simulink model "uGrid_1PH_hd_ATD2"  (R2018a)
settings: Solver=VariableStepAuto  StartTime=0.0  StopTime=0.8  FixedStep=1e-6  MaxStep=1e-4  RelTol=1e-3
PreLoadFcn:
  | SimulinkInit
InitFcn:
  | SimulinkInit
StopFcn:
  | EndingScript
values from neighbouring files (symbols this model uses):
  Ad = sysd.A    [SimulinkInit.m]
  Bd = sysd.B    [SimulinkInit.m]
  C1 = Cd(2,:)    [SimulinkInit.m]
  C10 = Cd(1,:)    [SimulinkInit.m]
  C11 = Cd(2,:)    [SimulinkInit.m]
  C12 = Cd(3,:)    [SimulinkInit.m]
  C2 = Cd(3,:)    [SimulinkInit.m]
  C3 = Cd(4,:)    [SimulinkInit.m]
  C4 = Cd(1,:)    [SimulinkInit.m]
  C5 = Cd(3,:)    [SimulinkInit.m]
  C6 = Cd(4,:)    [SimulinkInit.m]
  C7 = Cd(1,:)    [SimulinkInit.m]
  C8 = Cd(2,:)    [SimulinkInit.m]
  C9 = Cd(4,:)    [SimulinkInit.m]
  Cd = sysd.C    [SimulinkInit.m]
  T1 = 0.4    [parametros_BIO.m]
  T2 = 1    [parametros_BIO.m]
  T3 = 15    [parametros_BIO.m]
  T4 = 2.5    [parametros_BIO.m]
  T5 = 3.3    [parametros_BIO.m]
  Tao1 = 0.5    [SimulinkInit.m]
  tm = 1e-4    (= 0.0001)    [SimulinkInit.m]
undefined symbols (not defined in the file or in its folder): F1, F10, F11, F12, F2, F3, F4, F5, F6, F7, F8, F9, G, GF, H1, H10, H11, H12, H2, H3, H4, H5, H6, H7, H8, H9, Ion, K10U, K11U, K12U, K1U, K2U, K3U, K4U, K5U, K6U, K7U, K8U, K9U, Lithium, ss1, ss2, T10, T11, T12, T6, T7, T8, T9
libraries: powerlib x59, dsparch4 x17, truetime x12, powerlib_meascontrol x6, simulink x2, dspstat3 x2, dspfdesign x1, electricdrivelib x1
(part 3 of 3)

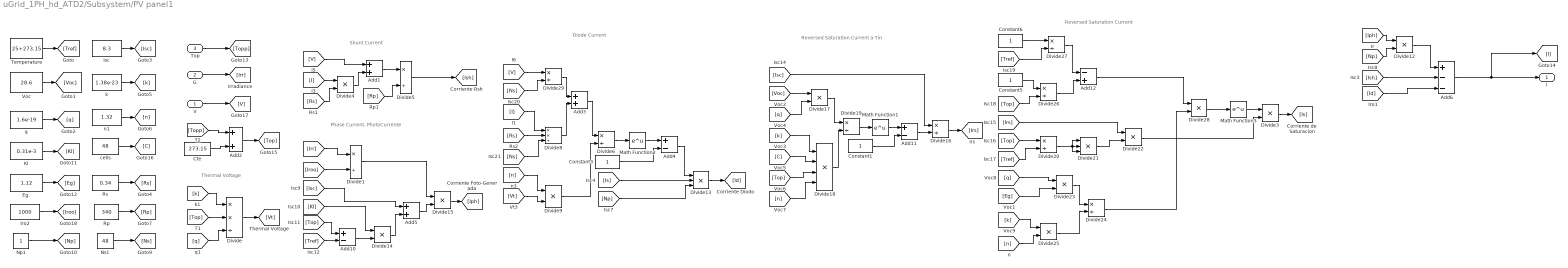
== system uGrid_1PH_hd_ATD2/Subsystem/PV panel1 ==
  note: Thermal Voltage
  note: Shunt Current
  note: Phase Current- PhotoCurrente
  note: Diode Current
  note: Reversed Saturation Current a Tin
  note: Reversed Saturation Current
  V : Inport
  G : Inport  Port=2
  Top : Inport  Port=3
  Add{1..3,5} (4 alike) : Sum
  Add10 : Sum  Inputs=+-
  Add11 : Sum  Inputs=+-
  Add12 : Sum  Inputs=-+
  Add4 : Sum  Inputs=+-
  Add6 : Sum  Inputs=+--
  Constant{1,3,5..6} (4 alike) : Constant
  Cte : Constant  Value=273.15
  Divide : Product  Inputs=**/
  Divide{1,5..6,16,19..20,24,26..27,29} (10 alike) : Product  Inputs=*/
  Divide{3..4,9,12,14..15,17,22..23,25,28} (11 alike) : Product  Inputs=**
  Divide13 : Product  Inputs=***
  Divide18 : Product  Inputs=****
  Divide21 : Product  Inputs=***
  Divide8 : Product  Inputs=**/
  Eg. : Constant  Value=1.12
  Iro2 : Constant  Value=1000
  Isc : Constant  Value=8.3
  KI : Constant  Value=0.31e-3
  Math Function1 : Math  SaturateOnIntegerOverflow=on
  Math Function2 : Math  SaturateOnIntegerOverflow=on
  Math Function3 : Math  SaturateOnIntegerOverflow=on
  Np1 : Constant
  Ns1 : Constant  Value=48
  Rp : Constant  Value=340
  Rs : Constant  Value=0.34
  Temperature : Constant  Value=25+273.15
  Voc : Constant  Value=28.6
  cells : Constant  Value=48
  k : Constant  Value=1.38e-23
  n1 : Constant  Value=1.32
  q : Constant  Value=1.6e-19
  I : Outport
  wires:
  Temperature/1 -> [Tref]
  Voc/1 -> [Voc]
  q/1 -> [q]
  Isc/1 -> [Isc]
  k/1 -> [k]
  n1/1 -> [n]
  [k] -> Divide/1
  [Top] -> Divide/2
  [q] -> Divide/3
  Divide/1 -> [Vt]
  Divide3/1 -> [Is]
  [Ish] -> Add6/2
  Add6/1 -> I/1, [I]
  [I] -> Divide8/1
  [Rs] -> Divide8/2
  Divide8/1 -> Add3/2
  [n] -> Divide9/1
  [Vt] -> Divide9/2
  Divide9/1 -> Divide6/2
  Add3/1 -> Divide6/1
  Divide6/1 -> Math Function2/1
  Math Function2/1 -> Add4/1
  Add4/1 -> Divide13/1
  [Is] -> Divide13/2
  Divide13/1 -> [Id]
  Divide4/1 -> Add1/2
  Add1/1 -> Divide5/1
  [Rp] -> Divide5/2
  Divide5/1 -> [Ish]
  [Rs] -> Divide4/2
  [I] -> Divide4/1
  KI/1 -> [KI]
  Eg./1 -> [Eg]
  [V] -> Add1/1
  [Np] -> Divide13/3
  [Iph] -> Divide12/1
  [Np] -> Divide12/2
  Divide12/1 -> Add6/1
  [Isc] -> Add5/1
  [Top] -> Add10/1
  [Tref] -> Add10/2
  Add10/1 -> Divide14/2
  [KI] -> Divide14/1
  [Voc] -> Divide17/1
  [q] -> Divide17/2
  [k] -> Divide18/1
  [C] -> Divide18/2
  [Top] -> Divide18/3
  [n] -> Divide18/4
  Divide17/1 -> Divide19/1
  Divide18/1 -> Divide19/2
  Divide19/1 -> Math Function1/1
  Constant1/1 -> Add11/2
  Math Function1/1 -> Add11/1
  Add11/1 -> Divide16/2
  Divide16/1 -> [Irs]
  [Tref] -> Divide20/2
  [Top] -> Divide20/1
  Divide20/1 -> Divide21/2, Divide21/1, Divide21/3
  Divide21/1 -> Divide22/2
  [Irs] -> Divide22/1
  [q] -> Divide23/1
  Divide23/1 -> Divide24/1
  [k] -> Divide25/1
  [n] -> Divide25/2
  Divide25/1 -> Divide24/2
  Constant5/1 -> Divide26/1
  [Top] -> Divide26/2
  Constant6/1 -> Divide27/1
  [Tref] -> Divide27/2
  Divide27/1 -> Add12/1
  Divide26/1 -> Add12/2
  Add12/1 -> Divide28/1
  Divide24/1 -> Divide28/2
  Divide28/1 -> Math Function3/1
  Divide29/1 -> Add3/1
  [Ns] -> Divide29/2
  [V] -> Divide29/1
  [Ns] -> Divide8/3
  Divide14/1 -> Add5/2
  Add5/1 -> Divide15/2
  Divide15/1 -> [Iph]
  V/1 -> [V]
  G/1 -> [Irr]
  Top/1 -> [Topp]
  cells/1 -> [C]
  [Id] -> Add6/3
  Cte/1 -> Add2/2
  Add2/1 -> [Top]
  [Topp] -> Add2/1
  [Irr] -> Divide1/1
  [Iroo] -> Divide1/2
  Divide1/1 -> Divide15/1
  Iro2/1 -> [Iroo]
  Rs/1 -> [Rs]
  Rp/1 -> [Rp]
  Ns1/1 -> [Ns]
  Np1/1 -> [Np]
  Constant3/1 -> Add4/2
  [Isc] -> Divide16/1
  Math Function3/1 -> Divide3/1
  Divide22/1 -> Divide3/2
  [Eg] -> Divide23/2

== system uGrid_1PH_hd_ATD2/1Ph_Inverter_bio/Subsystem/Steper1 ==
  In1 : Inport
  Product : Product
  Step : Step  Time=st_time  SampleTime=samp_f
  Out1 : Outport
  wires:
  Step/1 -> Product/2
  In1/1 -> Product/1
  Product/1 -> Out1/1

== system uGrid_1PH_hd_ATD2/1Ph_Inverter_bio/Subsystem/Steper3 ==
  In1 : Inport
  Product : Product
  Step : Step  Time=st_time  SampleTime=samp_f
  Out1 : Outport
  wires:
  Product/1 -> Out1/1
  In1/1 -> Product/1
  Step/1 -> Product/2

== system uGrid_1PH_hd_ATD2/1Ph_Inverter_diesel/Subsystem/Steper1 ==
  In1 : Inport
  Product : Product
  Step : Step  Time=st_time  SampleTime=samp_f
  Out1 : Outport
  wires:
  Product/1 -> Out1/1
  In1/1 -> Product/1
  Step/1 -> Product/2

== system uGrid_1PH_hd_ATD2/1Ph_Inverter_diesel/Subsystem/Steper3 ==
  In1 : Inport
  Product : Product
  Step : Step  Time=st_time  SampleTime=samp_f
  Out1 : Outport
  wires:
  Step/1 -> Product/2
  In1/1 -> Product/1
  Product/1 -> Out1/1

== matlab function uGrid_1PH_hd_ATD2/1Ph_Inverter_diesel/Subsystem/not_pwm ==
  data: u input; y output
function y = fcn(u)
%#codegen

if(u==0 || u<0)
    a=15;
else
    a=0;
end;

y = a;

== matlab function uGrid_1PH_hd_ATD2/1Ph_Inverter_bio/Subsystem/not_pwm ==
  data: u input; y output
function y = fcn(u)
%#codegen

if(u==0 || u<0)
    a=15;
else
    a=0;
end;

y = a;

== matlab function uGrid_1PH_hd_ATD2/LinearProg ==
  data: P_load input; Pbo output; P_e_alt input; kb input; kd input; PdMax input; PbMax input; Pdo output; P_e_alt_min input
function [Pbo, Pdo] = fcn(P_load, P_e_alt, kb, kd, PdMax, PbMax, P_e_alt_min)

% P_load es la potencia que se requiere en la carga.

% P_e_alt es la potencia estimada de generacion de las energias
% alternativas

% kb y kd son los pesos de las funcion de costo.

% las salidas son las potencias optimas para bio y diesel

Pb=0;
Pd=0;

D_P_e_alt = P_e_alt - P_e_alt_min % superaavit de energia alternativa.

flagDelt = 0;

if(D_P_e_alt >= P_load)
    flagDelt = 1;
end
   

if(flagDelt==0)
    P_trad = P_load - D_P_e_alt;
    % flag: variable que indica si tiene sentido evaluar los
    % if's que se encuentran mas adelante. es decir, si flag = 0 
    % despues del primer if entonces NO se le esta pidiendo al sistema
    % mas potencia de la que puede generar y portanto el problema de 
    % optimizacion lineal tiene sentido.
    % entonces 
    flag=0;

    if(P_trad>PdMax+PbMax)
        Pd=PdMax;
        Pb=PbMax;
        flag=1;
    end

    % si ambas energias tienen el mismo factor de costo.
    if(kd==kb && flag==0)
        Pb=P_trad/2;
        Pd=P_trad/2;
    end

    % si la energia diesel es mas cara que la biomasa.
    if(kd>kb && flag==0)
        if(P_trad<=PbMax)
            Pb=P_trad;
            Pd=0;
        else
            Pb=PbMax;
            Pd=P_trad-PbMax;
        end
    end

    % si la biomasa es mas cara que la diesel.
    if(kd<kb && flag==0)
        if(P_trad<=PdMax)
            Pd=P_trad;
            Pb=0;
        else
            Pd=PdMax;
            Pb=P_trad-PdMax;
        end
    end
end

Pbo=Pb;
Pdo=Pd;

== matlab function uGrid_1PH_hd_ATD2/MPC Controller/MPC_MatCalc1 ==
  data: ref input; PQ input; Hv output; F output; A output; lb output; ub output; lbA output; ubA output; Du input; MPCout input; G input; GF input
function [Hv, F, A, lb, ub, lbA, ubA] = MPC(ref, PQ, Du, MPCout, G, GF)

%%parametros del MPC


p = 100; % horizonte de prediccion
Nu = 100; % horizonte de control


%% Calculo de la salida de control.

H = G'*G+eye(2*Nu)*3000; % parte cuadratica del qp

ym = [ ones(p, 1)*PQ(1); ones(p, 1)*PQ(2) ]; % vector de la medida de tempearatura actual.

w = [ ones(p, 1)*ref(1); ones(p, 1)*ref(2) ]; % vector señal setpoint.

L = GF*Du+ym; % respuesta libre.

F = 2*(L-w)'*G; % parte lineal del problema qp.

A = zeros(1, 4*Nu*Nu);

lbA = zeros(1, 2*Nu);

ubA = zeros(1, 2*Nu);

Hv = M2V(H);

hip = HiBound(MPCout(1), 600, 10);
hiq = HiBound(MPCout(2), 5000, 1000);

lop = LowBound(MPCout(1), -100, -10);
loq = LowBound(MPCout(2), -100, -1000);

lb = [ones(1, Nu)*lop ones(1, Nu)*loq];
ub = [ones(1, Nu)*hip ones(1, Nu)*hiq];
end

% el control mpc implementado halla mediante programacion cuadratica
% los delta de u optimos deacuerdo a la funcion de coste. por este motivo
% es necesario implementar una logica adicional que permita limitar
% los valores de u (la salida) ya que estos no se manupilan directamente
% en el problema de programacion cuadratica.

% esta logica se implementan en las dos funciones locales que se encuentran
% a continuacion. una funcion define el limite superior y otra funcion para
% definir el limite inferior de los deltas de u deacuerdo al valor actual
% de u para asegurar que tanto los deltas de u como el valor de u esten
% limitados.
% esta funcion solo es correcta si max y Dmax son valores positivos.
function y = HiBound(X, max, Dmax)
    if(X>=0) % si la potencia X es positiva:
        if(max >= X)% si X no ha superado la potencia maxima:
            if(max-X >= Dmax) % si la distancia supera el cambio maximo deseado
                r = Dmax;
            else % si es menor al cambio maximo deseado
                r = max-X;
            end
        else % si X supera la potencia maxima deseada
            r = 0; % el delta maximo es 0 para que no se incremente mas.
        end
    else % si la potencia X es negativa, el incremento maximo es
        r = Dmax;
    end
    y = r;
end

% esta funcion para el lower bound se penso para trbajar con valores
% negativos. si min y Dmin no es negativo la funcion no funciona
% correctamente.
function y = LowBound(X, minv, Dmin)
    if(X<=0) % si la potencia X esta en el cuadrante inferior:
        if(minv <= X)% si X es mayor que la potencia minima:
            if(minv-X <= Dmin) % si la distancia supera el cambio maximo deseado
                r = Dmin;
            else % si es mayor al cambio maximo deseado
                r = minv-X;
            end
        else % si X es menor la potencia maxima deseada
            r = 0; % el delta maximo es 0 para que no se decremente mas.
        end
    else % si la potencia X es positiva, el decremento maximo es
        r = Dmin;
    end
    y = r;
end

== matlab function uGrid_1PH_hd_ATD2/MPC Controller/MPC_OutLogic1 ==
  data: MPCout output; duv input; Duv output
function [MPCout, Duv] = MPC_out_Logic(duv)

%%parametros del MPC
Nu = 100; % horizonte de control.


%% variables del MPC
persistent Du; % deltas de u 
persistent out; % salida actual del conrolador MPC.

if isempty(Du) % inicializacion de los deltas de uu
    Du = zeros(2*Nu, 1);
end

if isempty(out) % inicializaion de la salida del controlador MPC
    out = [0; 0];
end


du = [duv(1), duv(Nu+1)];


Du = [du(1); Du(1:Nu-1); du(2); Du(Nu+1:end-1)];% actualizar historial deltas de u.

out = [ out(1)+du(1); out(2)+du(2) ]; %calcular salida del controlador.

MPCout = out;
Duv = Du;

== matlab function uGrid_1PH_hd_ATD2/MPC Controller/MPC_MatCalc ==
  data: ref input; PQ input; Hv output; F output; A output; lb output; ub output; lbA output; ubA output; Du input; MPCout input; G input; GF input
function [Hv, F, A, lb, ub, lbA, ubA] = MPC(ref, PQ, Du, MPCout, G, GF)

%%parametros del MPC


p = 100; % horizonte de prediccion
Nu = 100; % horizonte de control


%% Calculo de la salida de control.

H = G'*G+eye(2*Nu)*3000; % parte cuadratica del qp

ym = [ ones(p, 1)*PQ(1); ones(p, 1)*PQ(2) ]; % vector de la medida de tempearatura actual.

w = [ ones(p, 1)*ref(1); ones(p, 1)*ref(2) ]; % vector señal setpoint.

L = GF*Du+ym; % respuesta libre.

F = 2*(L-w)'*G; % parte lineal del problema qp.

A = zeros(1, 4*Nu*Nu);

lbA = zeros(1, 2*Nu);

ubA = zeros(1, 2*Nu);

Hv = M2V(H);

hip = HiBound(MPCout(1), 600, 10);
hiq = HiBound(MPCout(2), 5000, 1000);

lop = LowBound(MPCout(1), -100, -10);
loq = LowBound(MPCout(2), -100, -1000);

lb = [ones(1, Nu)*lop ones(1, Nu)*loq];
ub = [ones(1, Nu)*hip ones(1, Nu)*hiq];
end

% el control mpc implementado halla mediante programacion cuadratica
% los delta de u optimos deacuerdo a la funcion de coste. por este motivo
% es necesario implementar una logica adicional que permita limitar
% los valores de u (la salida) ya que estos no se manupilan directamente
% en el problema de programacion cuadratica.

% esta logica se implementan en las dos funciones locales que se encuentran
% a continuacion. una funcion define el limite superior y otra funcion para
% definir el limite inferior de los deltas de u deacuerdo al valor actual
% de u para asegurar que tanto los deltas de u como el valor de u esten
% limitados.
% esta funcion solo es correcta si max y Dmax son valores positivos.
function y = HiBound(X, max, Dmax)
    if(X>=0) % si la potencia X es positiva:
        if(max >= X)% si X no ha superado la potencia maxima:
            if(max-X >= Dmax) % si la distancia supera el cambio maximo deseado
                r = Dmax;
            else % si es menor al cambio maximo deseado
                r = max-X;
            end
        else % si X supera la potencia maxima deseada
            r = 0; % el delta maximo es 0 para que no se incremente mas.
        end
    else % si la potencia X es negativa, el incremento maximo es
        r = Dmax;
    end
    y = r;
end

% esta funcion para el lower bound se penso para trbajar con valores
% negativos. si min y Dmin no es negativo la funcion no funciona
% correctamente.
function y = LowBound(X, minv, Dmin)
    if(X<=0) % si la potencia X esta en el cuadrante inferior:
        if(minv <= X)% si X es mayor que la potencia minima:
            if(minv-X <= Dmin) % si la distancia supera el cambio maximo deseado
                r = Dmin;
            else % si es mayor al cambio maximo deseado
                r = minv-X;
            end
        else % si X es menor la potencia maxima deseada
            r = 0; % el delta maximo es 0 para que no se decremente mas.
        end
    else % si la potencia X es positiva, el decremento maximo es
        r = Dmin;
    end
    y = r;
end

== matlab function uGrid_1PH_hd_ATD2/MPC Controller/MPC_OutLogic ==
  data: MPCout output; duv input; Duv output
function [MPCout, Duv] = MPC_out_Logic(duv)

%%parametros del MPC
Nu = 100; % horizonte de control.


%% variables del MPC
persistent Du; % deltas de u 
persistent out; % salida actual del conrolador MPC.

if isempty(Du) % inicializacion de los deltas de uu
    Du = zeros(2*Nu, 1);
end

if isempty(out) % inicializaion de la salida del controlador MPC
    out = [0; 0];
end


du = [duv(1), duv(Nu+1)];


Du = [du(1); Du(1:Nu-1); du(2); Du(Nu+1:end-1)];% actualizar historial deltas de u.

out = [ out(1)+du(1); out(2)+du(2) ]; %calcular salida del controlador.

MPCout = out;
Duv = Du;

== matlab function uGrid_1PH_hd_ATD2/1Ph_Inverter_bio1/not_pwm ==
  data: u input; y output
function y = fcn(u)
%#codegen

if(u==0 || u<0)
    a=15;
else
    a=0;
end;

y = a;

== matlab function uGrid_1PH_hd_ATD2/BioMassGenerator/Subsystem1/MATLAB Function ==
  data: w input; Pe input; Tm output
function Tm = fcn(w, Pe)

max_torq=30000;

if w>0
    Tm = Pe/w;
else
    Tm = max_torq;
end

== matlab function uGrid_1PH_hd_ATD2/LinearProg1 ==
  data: Q_load input; Qbo output; Q_e_alt input; kb input; kd input; QdMax input; QbMax input; Qdo output; Q_e_alt_min input
function [Qbo, Qdo] = fcn(Q_load, Q_e_alt, kb, kd, QdMax, QbMax, Q_e_alt_min)

% Q_load es la Qotencia que se requiere en la carga.

% Q_e_alt es la Qotencia estimada de generacion de las energias
% alternativas

% kb y kd son los Qesos de las funcion de costo.

% las salidas son las Qotencias oQtimas Qara bio y diesel

Qb=0;
Qd=0;

D_Q_e_alt = Q_e_alt - Q_e_alt_min % suQeraavit de energia alternativa.

flagDelt = 0;

if(D_Q_e_alt >= Q_load)
    flagDelt = 1;
end
   

if(flagDelt==0)
    Q_trad = Q_load - D_Q_e_alt;
    % flag: variable que indica si tiene sentido evaluar los
    % if's que se encuentran mas adelante. es decir, si flag = 0 
    % desQues del Qrimer if entonces NO se le esta Qidiendo al sistema
    % mas Qotencia de la que Quede generar y Qortanto el Qroblema de 
    % oQtimizacion lineal tiene sentido.
    % entonces 
    flag=0;

    if(Q_trad>QdMax+QbMax)
        Qd=QdMax;
        Qb=QbMax;
        flag=1;
    end

    % si ambas energias tienen el mismo factor de costo.
    if(kd==kb && flag==0)
        Qb=Q_trad/2;
        Qd=Q_trad/2;
    end

    % si la energia diesel es mas cara que la biomasa.
    if(kd>kb && flag==0)
        if(Q_trad<=QbMax)
            Qb=Q_trad;
            Qd=0;
        else
            Qb=QbMax;
            Qd=Q_trad-QbMax;
        end
    end

    % si la biomasa es mas cara que la diesel.
    if(kd<kb && flag==0)
        if(Q_trad<=QdMax)
            Qd=Q_trad;
            Qb=0;
        else
            Qd=QdMax;
            Qb=Q_trad-QdMax;
        end
    end
end

Qbo=Qb;
Qdo=Qd;

== matlab function uGrid_1PH_hd_ATD2/FRACASO/MATLAB Function4 ==
  data: r input; rol output; r1 input
function rol = fcn(r,r1)%u1,u2,ym1,ym2)
Th_det = 6.5e-8;
Th_det=0.1;  %2.5

m=r-r1;
if m>0
    Th_det=0.1;  %2.5
elseif m<0 && r<=0.1
    Th_det=0.9; 
end


% sys=tf(1,[0.001 1]);


if r >=Th_det
    rol=1;
else
    rol=0;
end

== matlab function uGrid_1PH_hd_ATD2/FRACASO/MATLAB Function3 ==
  data: y_hat input; rol output; y_m input; norm_rd output; tiempo input
function [rol,norm_rd] = fcn(y_hat,y_m,tiempo)%u1,u2,ym1,ym2)
Th_det = 6.5e-8;
Th_det=0.07;%2.3e-2; %Funciona bien si los pulsos no estan tan separados
Th_det_up=1;  %2.5 2.25
Th_det_down=-1;
if tiempo >=0.0015 && tiempo <=0.35
    Th_det_up=2.23e-2;  %2.5 2.25
    Th_det_down=3e-4;
else
    Th_det_up=2.25e-2;  %2.5 2.25
    Th_det_down=3e-3;
end
% Th_det=38;
% yol=[u1 ; u2];
% ym=[ym1 ; ym2];

rd1=(y_hat(1)-y_m(1))/100;%200;
rd2=(y_hat(2)-y_m(2))/120;%500;
rd3=(y_hat(3)-y_m(3))/400;%1300; 
rd4=(y_hat(4)-y_m(4))/500;

% rd=y_hat-y_m;
rd=[rd1 rd2 rd3 rd4];
norm_rd=sqrt(sum(rd.^2));
% sys=tf(1,[0.001 1]);


if norm_rd >=Th_det%Th_det_up && norm_rd <=Th_det_down
    rol=1;
else
    rol=0;
end

== matlab function uGrid_1PH_hd_ATD2/FRACASO/MATLAB Function1 ==
  data: y_hat input; y output; t input
function y = fcn(y_hat,t)%u1,u2,ym1,ym2)
if t<=0.33
    y1=y_hat(1)*1;%0.92;
    y2=y_hat(2)*1;
    y3=y_hat(3)*0.77;%1.1; 0.71 0.77 +28
%     if y3<0
%         y3=y3+11;
%     end
    y4=y_hat(4)*1;%y_hat(4)*1;
    


else
    y1=y_hat(1)*1;%0.92;
    y2=y_hat(2)*1;
    y3=y_hat(3)*0.65;%1.1; 0.65
    y4=y_hat(4)*1;%y_hat(4)*1;
end

y=[y1 y2 y3 y4];
% if norm_rd >=Th_det
%     rol=1;
% else
%     rol=0;
% end

== matlab function uGrid_1PH_hd_ATD2/FRACASO/MATLAB Function2 ==
  data: r input; y output
function y = fcn(r)%u1,u2,ym1,ym2)

r1=r(1)/2000;%200;
r2=r(2)/2000;%500;
r3=r(3)/2000;%1300;
r4=r(4)/2000;
y=[r1 r2 r3 r4];
% if norm_rd >=Th_det
%     rol=1;
% else
%     rol=0;
% end

== matlab function uGrid_1PH_hd_ATD2/MeasureNode_I2/MATLAB Function ==
  data: u1 input; y output; u2 input
function y = fcn(u1,u2)
if u1>=0.4 && u1<=0.45%u1>=1000
    y=u2+u2*0.25;
else
    y = u2;

end

== matlab function uGrid_1PH_hd_ATD2/MeasureNode_I4/MATLAB Function ==
  data: u1 input; y output; u2 input
function y = fcn(u1,u2)
if u1>=0.6 && u1<=0.66%u1>=1000
    y=u2+u2*0.3;
else
    y = u2;

end

== matlab function uGrid_1PH_hd_ATD2/MeasureNode_I3/MATLAB Function ==
  data: u1 input; y output; u2 input
function y = fcn(u1,u2)
if u1>=0.10 && u1<=0.2%u1>=1000
    y=u2+u2*0.3;
else
    y = u2;

end

== matlab function uGrid_1PH_hd_ATD2/MeasureNode_I1/MATLAB Function ==
  data: u1 input; y output; u2 input
function y = fcn(u1,u2)
if u1>=0.50 && u1<=0.55%u1>=1000
    y=u2-u2*0.25;
else
    y = u2;

end

== matlab function uGrid_1PH_hd_ATD2/FRACASO/MATLAB Function5 ==
  data: r input; rol output; x1 input; xp output; x input; m output
function [rol,xp,m]= fcn(r,x1,x)%u1,u2,ym1,ym2)
Th_det = 6.5e-8;
Th_det=0.1;  %2.5

tao1=0.0025;
tao2=0.0525;
m=x-x1;

% xp= r/tao1-x/tao1;

xp=0;

if m>0
    xp= r/tao1-x/tao1;
    Th_det=0.1;  %2.5
elseif m<0 && x<=0.8
    xp= r/tao2-x/tao2;
    Th_det=0.9; 
end



% sys=tf(1,[0.001 1]);


if x >=Th_det
    rol=1;
else
    rol=0;
end

== matlab function uGrid_1PH_hd_ATD2/FRACASO/MATLAB Function6 ==
  data: r input; rol output; r1 input
function rol = fcn(r,r1)%u1,u2,ym1,ym2)
Th_det = 6.5e-8;
Th_det=0.1;  %2.5

m=r-r1;
if m>0
    Th_det=0.1;  %2.5
elseif m<0 && r<=0.1
    Th_det=0.9; 
end


% sys=tf(1,[0.001 1]);


if r >=Th_det
    rol=1;
else
    rol=0;
end

== matlab function uGrid_1PH_hd_ATD2/FRACASO/MATLAB Function7 ==
  data: r input; rol output; r1 input; Th_det output
function [rol,Th_det] = fcn(r,r1)%u1,u2,ym1,ym2)
% Th_det = 6.5e-8;
Th_det=0.08;  %2.5

m=r-r1;
if m>0
    Th_det=0.07;%0.1;  %2.5
elseif m<0 && r<=0.007
    Th_det=0.9; 
end


% sys=tf(1,[0.001 1]);


if r >=Th_det
    rol=1;
else
    rol=0;
end

== matlab function uGrid_1PH_hd_ATD2/FRACASO/MATLAB Function10 ==
  data: x_hat1 input; v1 output; x_hat2 input; ruo1 input; rol input
function v1 = fcn(x_hat1,x_hat2,ruo1,rol)

% yol=[u1 ; u2];
% ym=[ym1 ; ym2];
 C1=[1     0     0];
 v1=C1*(x_hat1-x_hat2)*ruo1*rol;

== matlab function uGrid_1PH_hd_ATD2/FRACASO/MATLAB Function11 ==
  data: x_hat1 input; v2 output; x_hat2 input; ruo2 input; rol input
function v2 = fcn(x_hat1,x_hat2,ruo2,rol)

% yol=[u1 ; u2];
% ym=[ym1 ; ym2];
 C2=[0     1     0];
 v2=C2*(x_hat2-x_hat1)*ruo2*rol;

== matlab function uGrid_1PH_hd_ATD2/FRACASO/MATLAB Function8 ==
  data: ya input; ruo1 output; ym input
function ruo1 = fcn(ya,ym)
Th_uio_on = 3e-3;
Th_uio_off = 1e-5;


Th_uio_on = 6e-3;


% yol=[u1 ; u2];
% ym=[ym1 ; ym2];

% rd1=ya1-ym1;
% rd2=ya2-ym2;

% ya=[ya(1:3)y(5)];
r=ya-ym;

if abs(r(1))  >= Th_uio_on && abs(r(2))  <= Th_uio_off && abs(r(3))  <= Th_uio_off && abs(r(4))  <= Th_uio_off
    ruo1=1;
else
    ruo1=0;
end

== matlab function uGrid_1PH_hd_ATD2/FRACASO/MATLAB Function9 ==
  data: ya input; ruo2 output; ym input
function ruo2 = fcn(ya,ym)
Th_uio_on = 3e-3;
Th_uio_off = 1e-5;


Th_uio_on = 6e-3;


% yol=[u1 ; u2];
% ym=[ym1 ; ym2];

% rd1=ya1-ym1;
% rd2=ya2-ym2;

% ya=[ya(1:3)y(5)];
r=ya-ym;

if abs(r(1))  >= Th_uio_on && abs(r(2))  <= Th_uio_off && abs(r(3))  <= Th_uio_off && abs(r(4))  <= Th_uio_off
    ruo2=1;
else
    ruo2=0;
end

== matlab function uGrid_1PH_hd_ATD2/FRACASO/MATLAB Function12 ==
  data: ya input; ruo3 output; ym input
function ruo3 = fcn(ya,ym)
Th_uio_on = 3e-3;
Th_uio_off = 1e-5;


Th_uio_on = 6e-3;


% yol=[u1 ; u2];
% ym=[ym1 ; ym2];

% rd1=ya1-ym1;
% rd2=ya2-ym2;

% ya=[ya(1:3)y(5)];
r=ya-ym;

if abs(r(1))  >= Th_uio_on && abs(r(2))  <= Th_uio_off && abs(r(3))  <= Th_uio_off && abs(r(4))  <= Th_uio_off
    ruo3=1;
else
    ruo3=0;
end

== matlab function uGrid_1PH_hd_ATD2/FRACASO/MATLAB Function13 ==
  data: ya input; ruo4 output; ym input
function ruo4 = fcn(ya,ym)
Th_uio_on = 3e-3;
Th_uio_off = 1e-5;


Th_uio_on = 6e-3;


% yol=[u1 ; u2];
% ym=[ym1 ; ym2];

% rd1=ya1-ym1;
% rd2=ya2-ym2;

% ya=[ya(1:3)y(5)];
r=ya-ym;

if abs(r(1))  >= Th_uio_on && abs(r(2))  <= Th_uio_off && abs(r(3))  <= Th_uio_off && abs(r(4))  <= Th_uio_off
    ruo4=1;
else
    ruo4=0;
end

== matlab function uGrid_1PH_hd_ATD2/MATLAB Function1 ==
  data: y_hat input; y output; t input
function y = fcn(y_hat,t)%u1,u2,ym1,ym2)
if y_hat(3)>0
    y_hat(3)=y_hat(3)*1.38;
    %     y_hat(3)=y_hat(3)+10;
end

% if t<=0.33
%     y1=y_hat(1)*1;%0.92;
%     y2=y_hat(2)*1;
%     y3=y_hat(3)*1;%1.1; 0.71 0.77 +28
% %     if y3<0
% %         y3=y3+11;
% %     end
%     y4=y_hat(4)*1;%y_hat(4)*1;
%
%
%
% else
%     y1=y_hat(1)*1;%0.92;
%     y2=y_hat(2)*1;
%     y3=y_hat(3)*0.4;%1.1; 0.65; 0.5
%     y4=y_hat(4)*1;%y_hat(4)*1;
% end
if t<=0.33
    y1=y_hat(1)*0.85;
    y2=y_hat(2)*0.8; %0.85
    y3=y_hat(3)*0.57; %0.6
    y4=y_hat(4)*0.88; %0.9
else
    y1=y_hat(1)*0.98;
    y2=y_hat(2)*1.16; %1.13  1.16
    y3=y_hat(3)*0.45; %0.5
    y4=y_hat(4);
    
end

y=[y1 y2 y3 y4];
% if norm_rd >=Th_det
%     rol=1;
% else
%     rol=0;
% end

== matlab function uGrid_1PH_hd_ATD2/MATLAB Function2 ==
  data: r input; y output
function y = fcn(r)%u1,u2,ym1,ym2)

r1=r(1)/2000;%200;
r2=r(2)/2000;%500;
r3=r(3)/2000;%1300;
r4=r(4)/2000;
y=[r1 r2 r3 r4];
% if norm_rd >=Th_det
%     rol=1;
% else
%     rol=0;
% end

== matlab function uGrid_1PH_hd_ATD2/MATLAB Function3 ==
  data: y_hat input; rol output; y_m input; norm_rd output; tiempo input
function [rol,norm_rd] = fcn(y_hat,y_m,tiempo)%u1,u2,ym1,ym2)
Th_det = 6.5e-8;
Th_det=0.07;%2.3e-2; %Funciona bien si los pulsos no estan tan separados
Th_det_up=1;  %2.5 2.25
Th_det_down=-1;
if tiempo >=0.0015 && tiempo <=0.35
    Th_det_up=2.23e-2;  %2.5 2.25
    Th_det_down=3e-4;
else
    Th_det_up=2.25e-2;  %2.5 2.25
    Th_det_down=3e-3;
end
% Th_det=38;
% yol=[u1 ; u2];
% ym=[ym1 ; ym2];

rd1=(y_hat(1)-y_m(1))/100;%200;
rd2=(y_hat(2)-y_m(2))/120;%500;
rd3=(y_hat(3)-y_m(3))/400;%1300; 
rd4=(y_hat(4)-y_m(4))/500;

% rd=y_hat-y_m;
rd=[rd1 rd2 rd3 rd4];
norm_rd=sqrt(sum(rd.^2));
% sys=tf(1,[0.001 1]);


if norm_rd >=Th_det%Th_det_up && norm_rd <=Th_det_down
    rol=1;
else
    rol=0;
end

== matlab function uGrid_1PH_hd_ATD2/MATLAB Function ==
  data: u input; y output; t input
function y = fcn(u,t)
y1=u(1);
y2=u(2);
if t<=0.33
    y3=u(3)*0.69;%*0.52;
else
    y3=u(3)*0.52;
end
y4=u(4);
y5=u(5);
y = [y1 y2 y3 y4 y5];

== matlab function uGrid_1PH_hd_ATD2/MATLAB Function7 ==
  data: r input; rol output; r1 input; Th_det output
function [rol,Th_det] = fcn(r,r1)%u1,u2,ym1,ym2)
% Th_det = 6.5e-8;
Th_det=0.08;  %2.5

m=r-r1;
if m>0
    Th_det=0.07;%0.1;  %2.5
elseif m<0 && r<=0.007
    Th_det=0.9; 
end


% sys=tf(1,[0.001 1]);


if r >=Th_det
    rol=1;
else
    rol=0;
end

== matlab function uGrid_1PH_hd_ATD2/MATLAB Function12 ==
  data: ya input; ruo3 output; ym input
function ruo3 = fcn(ya,ym)
Th_uio_on = 3e-3;
Th_uio_off = 1e-5;


Th_uio_on = 6e-3;


% yol=[u1 ; u2];
% ym=[ym1 ; ym2];

% rd1=ya1-ym1;
% rd2=ya2-ym2;

% ya=[ya(1:3)y(5)];
r=ya-ym;

if abs(r(1))  >= Th_uio_on && abs(r(2))  <= Th_uio_off && abs(r(3))  <= Th_uio_off && abs(r(4))  <= Th_uio_off
    ruo3=1;
else
    ruo3=0;
end

== matlab function uGrid_1PH_hd_ATD2/MATLAB Function13 ==
  data: ya input; ruo4 output; ym input
function ruo4 = fcn(ya,ym)
Th_uio_on = 3e-3;
Th_uio_off = 1e-5;


Th_uio_on = 6e-3;


% yol=[u1 ; u2];
% ym=[ym1 ; ym2];

% rd1=ya1-ym1;
% rd2=ya2-ym2;

% ya=[ya(1:3)y(5)];
r=ya-ym;

if abs(r(1))  >= Th_uio_on && abs(r(2))  <= Th_uio_off && abs(r(3))  <= Th_uio_off && abs(r(4))  <= Th_uio_off
    ruo4=1;
else
    ruo4=0;
end

== matlab function uGrid_1PH_hd_ATD2/MATLAB Function15 ==
  data: ya input; ruo4 output; ym input
function ruo4 = fcn(ya,ym)
Th_uio_on = 3e-3;
Th_uio_off = 1e-5;


Th_uio_on = 6e-3;


% yol=[u1 ; u2];
% ym=[ym1 ; ym2];

% rd1=ya1-ym1;
% rd2=ya2-ym2;

% ya=[ya(1:3)y(5)];
r=ya-ym;

if abs(r(1))  >= Th_uio_on && abs(r(2))  <= Th_uio_off && abs(r(3))  <= Th_uio_off && abs(r(4))  <= Th_uio_off
    ruo4=1;
else
    ruo4=0;
end

== matlab function uGrid_1PH_hd_ATD2/MATLAB Function16 ==
  data: ya input; ruo4 output; ym input
function ruo4 = fcn(ya,ym)
Th_uio_on = 3e-3;
Th_uio_off = 1e-5;


Th_uio_on = 6e-3;


% yol=[u1 ; u2];
% ym=[ym1 ; ym2];

% rd1=ya1-ym1;
% rd2=ya2-ym2;

% ya=[ya(1:3)y(5)];
r=ya-ym;

if abs(r(1))  >= Th_uio_on && abs(r(2))  <= Th_uio_off && abs(r(3))  <= Th_uio_off && abs(r(4))  <= Th_uio_off
    ruo4=1;
else
    ruo4=0;
end

== matlab function uGrid_1PH_hd_ATD2/MATLAB Function17 ==
  data: ya input; ruo4 output; ym input
function ruo4 = fcn(ya,ym)
Th_uio_on = 3e-3;
Th_uio_off = 1e-5;


Th_uio_on = 6e-3;


% yol=[u1 ; u2];
% ym=[ym1 ; ym2];

% rd1=ya1-ym1;
% rd2=ya2-ym2;

% ya=[ya(1:3)y(5)];
r=ya-ym;

if abs(r(1))  >= Th_uio_on && abs(r(2))  <= Th_uio_off && abs(r(3))  <= Th_uio_off && abs(r(4))  <= Th_uio_off
    ruo4=1;
else
    ruo4=0;
end

== matlab function uGrid_1PH_hd_ATD2/MATLAB Function18 ==
  data: ya input; ruo4 output; ym input
function ruo4 = fcn(ya,ym)
Th_uio_on = 3e-3;
Th_uio_off = 1e-5;


Th_uio_on = 6e-3;


% yol=[u1 ; u2];
% ym=[ym1 ; ym2];

% rd1=ya1-ym1;
% rd2=ya2-ym2;

% ya=[ya(1:3)y(5)];
r=ya-ym;

if abs(r(1))  >= Th_uio_on && abs(r(2))  <= Th_uio_off && abs(r(3))  <= Th_uio_off && abs(r(4))  <= Th_uio_off
    ruo4=1;
else
    ruo4=0;
end

== matlab function uGrid_1PH_hd_ATD2/MATLAB Function19 ==
  data: ya input; ruo4 output; ym input
function ruo4 = fcn(ya,ym)
Th_uio_on = 3e-3;
Th_uio_off = 1e-5;


Th_uio_on = 6e-3;


% yol=[u1 ; u2];
% ym=[ym1 ; ym2];

% rd1=ya1-ym1;
% rd2=ya2-ym2;

% ya=[ya(1:3)y(5)];
r=ya-ym;

if abs(r(1))  >= Th_uio_on && abs(r(2))  <= Th_uio_off && abs(r(3))  <= Th_uio_off && abs(r(4))  <= Th_uio_off
    ruo4=1;
else
    ruo4=0;
end

== matlab function uGrid_1PH_hd_ATD2/MATLAB Function20 ==
  data: ya input; ruo4 output; ym input
function ruo4 = fcn(ya,ym)
Th_uio_on = 3e-3;
Th_uio_off = 1e-5;


Th_uio_on = 6e-3;


% yol=[u1 ; u2];
% ym=[ym1 ; ym2];

% rd1=ya1-ym1;
% rd2=ya2-ym2;

% ya=[ya(1:3)y(5)];
r=ya-ym;

if abs(r(1))  >= Th_uio_on && abs(r(2))  <= Th_uio_off && abs(r(3))  <= Th_uio_off && abs(r(4))  <= Th_uio_off
    ruo4=1;
else
    ruo4=0;
end

== matlab function uGrid_1PH_hd_ATD2/MATLAB Function21 ==
  data: ya input; ruo4 output; ym input
function ruo4 = fcn(ya,ym)
Th_uio_on = 3e-3;
Th_uio_off = 1e-5;


Th_uio_on = 6e-3;


% yol=[u1 ; u2];
% ym=[ym1 ; ym2];

% rd1=ya1-ym1;
% rd2=ya2-ym2;

% ya=[ya(1:3)y(5)];
r=ya-ym;

if abs(r(1))  >= Th_uio_on && abs(r(2))  <= Th_uio_off && abs(r(3))  <= Th_uio_off && abs(r(4))  <= Th_uio_off
    ruo4=1;
else
    ruo4=0;
end

== matlab function uGrid_1PH_hd_ATD2/MATLAB Function22 ==
  data: ya input; ruo4 output; ym input
function ruo4 = fcn(ya,ym)
Th_uio_on = 3e-3;
Th_uio_off = 1e-5;


Th_uio_on = 6e-3;


% yol=[u1 ; u2];
% ym=[ym1 ; ym2];

% rd1=ya1-ym1;
% rd2=ya2-ym2;

% ya=[ya(1:3)y(5)];
r=ya-ym;

if abs(r(1))  >= Th_uio_on && abs(r(2))  <= Th_uio_off && abs(r(3))  <= Th_uio_off && abs(r(4))  <= Th_uio_off
    ruo4=1;
else
    ruo4=0;
end

== matlab function uGrid_1PH_hd_ATD2/MATLAB Function24 ==
  data: u input; y output; t input
function y = fcn(u,t)
y1=u(1);
y2=u(2);
if t>0.33
    y2=u(2)*1.31;%*0.52;
    y5=u(5)*1.55;
else
    y2=u(2);
    
    y5=u(5)*1.39;
    
end
y3=u(3);
y4=u(4);


y = [y1 y2 y3 y4 y5];

== matlab function uGrid_1PH_hd_ATD2/MATLAB Function25 ==
  data: u input; y output; t input
function y = fcn(u,t)
y1=u(1);
y2=u(2);
if t>0.33
    y3=u(3)*0.54+5;
    y5=u(5)*1.15;
else
    y3=u(3)*0.7;
    
    y5=u(5);
    
end

y4=u(4);


y = [y1 y2 y3 y4 y5];

== matlab function uGrid_1PH_hd_ATD2/MATLAB Function26 ==
  data: u input; y output; t input
function y = fcn(u,t)
y1=u(1);
y2=u(2);
if t>0.33
    y2=u(2)*1.32;
    y5=u(5)*1.52;
else
    y2=u(2);
    y5=u(5)*1.4;
      
end
y3=u(3);
y4=u(4);



y = [y1 y2 y3 y4 y5];

== matlab function uGrid_1PH_hd_ATD2/MATLAB Function27 ==
  data: u input; y output; t input
function y = fcn(u,t)
y1=u(1);
y2=u(2);
% if t>0.33
%     y2=u(2)*1.32;
%     y5=u(5)*1.52;
% else
%     y2=u(2);
%     y5=u(5)*1.4;
      
% end
y3=u(3);
y4=u(4);
y5=u(5);



y = [y1 y2 y3 y4 y5];

== matlab function uGrid_1PH_hd_ATD2/MATLAB Function28 ==
  data: u input; y output; t input
function y = fcn(u,t)
y1=u(1);
y2=u(2);
if t>0.33
    y3=u(3)*0.54+5;
    y5=u(5)*1.14;
else
    y3=u(3)*0.7;
    y5=u(5);
      
end
% y3=u(3);
y4=u(4);



y = [y1 y2 y3 y4 y5];

== matlab function uGrid_1PH_hd_ATD2/MATLAB Function29 ==
  data: u input; y output; t input
function y = fcn(u,t)
y1=u(1);
y2=u(2);
if t>0.33
    y3=u(3)*0.54;
%     y5=u(5)*1.14;
else
    y3=u(3)*0.7;
%     y5=u(5);
      
end
% y3=u(3);
y4=u(4);
y5=u(5);



y = [y1 y2 y3 y4 y5];

== matlab function uGrid_1PH_hd_ATD2/MATLAB Function30 ==
  data: u input; y output; t input
function y = fcn(u,t)
y1=u(1);
y2=u(2);
% if t>0.33
%     y3=u(3)*0.54;
% %     y5=u(5)*1.14;
% else
%     y3=u(3)*0.7;
% %     y5=u(5);
%       
% end
y3=u(3);
y4=u(4);
y5=u(5);



y = [y1 y2 y3 y4 y5];

== matlab function uGrid_1PH_hd_ATD2/MATLAB Function31 ==
  data: u input; y output; t input
function y = fcn(u,t)
y1=u(1);
y2=u(2);
if t>0.33
    y3=u(3)*0.54;
    y5=u(5)*1.13;
else
    y3=u(3)*0.7;
    y5=u(5);
      
end
% y3=u(3);
y4=u(4);
% y5=u(5);



y = [y1 y2 y3 y4 y5];

== matlab function uGrid_1PH_hd_ATD2/MATLAB Function32 ==
  data: u input; y output; t input
function y = fcn(u,t)
y1=u(1); %-5  +5

if t>0.33
    y2=u(2)*1.27;
    
    y5=u(5)*1.47;
else
    y2=u(2);
    
    y5=u(5)*1.34;
    
end
y3=u(3);
y4=u(4);
% y5=u(5);



y = [y1 y2 y3 y4 y5];

== matlab function uGrid_1PH_hd_ATD2/MATLAB Function33 ==
  data: u input; y output; t input
function y = fcn(u,t)
y1=u(1)-10;
y2=u(2);
if t>0.33
    y3=u(3)*0.54;
%     y5=u(5)*1.14;
else
    y3=u(3)*0.7;
%     y5=u(5);
      
end
% y3=u(3);
y4=u(4);
y5=u(5);



y = [y1 y2 y3 y4 y5];

== matlab function uGrid_1PH_hd_ATD2/MATLAB Function34 ==
  settings: updateMethod=DISCRETE
  data: dr input; r output; t input
function r   = fcn(dr,t)
persistent a
if isempty(a)
    a=1;
       
end
if t<=0.33
    th=2.5e4;
%     v=2;
else
    th=4e4;
%     v=3;
end

r=0;
if a==2
    r=1;
end
% ra=r;

if abs(dr(2))>th
    r=1;
    a=a+1;
%     if v==0
%         v=1;
elseif abs(dr(2))>th && a==2
    r=0;
    a=1;
end


%     
% else
%     r=0;
% % elseif abs(dr(1))>=th
% %     r=0;
% %     v=0;
% end

== matlab function uGrid_1PH_hd_ATD2/MATLAB Function35 ==
  settings: updateMethod=DISCRETE
  data: dr input; r output; t input
function r   = fcn(dr,t)
persistent a
if isempty(a)
    a=1;
       
end
if t<=0.33
    th=6.5e4;
%     v=2;
else
    th=8e4;
%     v=3;
end

r=0;
if a==2
    r=1;
end
% ra=r;

if abs(dr(3))>th
    r=1;
    a=a+1;
%     if v==0
%         v=1;
elseif abs(dr(3))>th && a==2
    r=0;
    a=1;
end


%     
% else
%     r=0;
% % elseif abs(dr(1))>=th
% %     r=0;
% %     v=0;
% end

== matlab function uGrid_1PH_hd_ATD2/MATLAB Function37 ==
  settings: updateMethod=DISCRETE
  data: dr input; r output; t input
function r   = fcn(dr,t)
persistent a
if isempty(a)
    a=1;
       
end
if t<=0.33
    th=2e4;
%     v=2;
else
    th=4e4;
%     v=3;
end

r=0;
if a==2
    r=1;
end
% ra=r;

if abs(dr(1))>th
    r=1;
    a=a+1;
%     if v==0
%         v=1;
elseif abs(dr(1))>th && a==2
    r=0;
    a=1;
end


%     
% else
%     r=0;
% % elseif abs(dr(1))>=th
% %     r=0;
% %     v=0;
% end

== matlab function uGrid_1PH_hd_ATD2/MATLAB Function8 ==
  data: ya input; ruo1 output; ym input
function ruo1 = fcn(ya,ym)
Th_uio_on = 3e-3;
Th_uio_off = 1e-5;


Th_uio_on = 6e-3;


% yol=[u1 ; u2];
% ym=[ym1 ; ym2];

% rd1=ya1-ym1;
% rd2=ya2-ym2;

% ya=[ya(1:3)y(5)];
r=ya-ym;

if abs(r(1))  >= Th_uio_on && abs(r(2))  <= Th_uio_off && abs(r(3))  <= Th_uio_off && abs(r(4))  <= Th_uio_off
    ruo1=1;
else
    ruo1=0;
end

== matlab function uGrid_1PH_hd_ATD2/MATLAB Function9 ==
  data: ya input; ruo2 output; ym input
function ruo2 = fcn(ya,ym)
Th_uio_on = 3e-3;
Th_uio_off = 1e-5;


Th_uio_on = 6e-3;


% yol=[u1 ; u2];
% ym=[ym1 ; ym2];

% rd1=ya1-ym1;
% rd2=ya2-ym2;

% ya=[ya(1:3)y(5)];
r=ya-ym;

if abs(r(1))  >= Th_uio_on && abs(r(2))  <= Th_uio_off && abs(r(3))  <= Th_uio_off && abs(r(4))  <= Th_uio_off
    ruo2=1;
else
    ruo2=0;
end
